simulink model "RATE_ADAPTIVE"  (R2020a)
settings: Solver=FixedStepAuto  StartTime=0.0  StopTime=10.0  FixedStep=1e-3  RelTol=1e-3  EnableMultiTasking=on
undefined symbols (not defined in the file): a, b, c, D0, D1, D10, D11, D12, D13, D2, D3, D4, D5, D6, D7, D8, D9, PTA0, PTA1, PTA2, PTB23, PTB9, PTC16, PTC17, PTC2, PTC3, PTC4, PTD0, PTD1, PTD2, PTD3
libraries: frdmk64flib x16, dspstat3 x1, hdlsllib x1
settings Model: ExtModeTrigDuration=5  Creator=marry  LastModifiedBy=marry
settings OptimizationCC: EnhancedBackFolding=on  PassReuseOutputArgsAs=Individual arguments  ZeroExternalMemoryAtStartup=off  ZeroInternalMemoryAtStartup=off  MaxStackSize=64  OptimizeBlockOrder=speed  DifferentSizesBufferReuse=on  OptimizationCustomize=off  EfficientTunableParamExpr=on
settings DebuggingCC: ParameterTunabilityLossMsg=error
settings HardwareCC: ProdBitPerPointer=32  ProdBitPerSizeT=32  ProdBitPerPtrDiffT=32  ProdLargestAtomicInteger=Long  ProdLargestAtomicFloat=Double  ProdWordSize=32  ProdHWDeviceType=ARM Compatible->ARM Cortex
settings SFSimCC: MATLABDynamicMemAlloc=off
settings RTWCC: SystemTargetFile=ert.tlc  HardwareBoard=NXP FRDM-K64F  TemplateMakefile=ert_default_tmf  Toolchain=GNU Tools for ARM Embedded Processors
settings CodeAppCC: ForceParamTrailComments=on  IgnoreCustomStorageClasses=off  OperatorAnnotations=on  SimulinkDataObjDesc=on  SFDataObjDesc=on  InsertBlockDesc=on

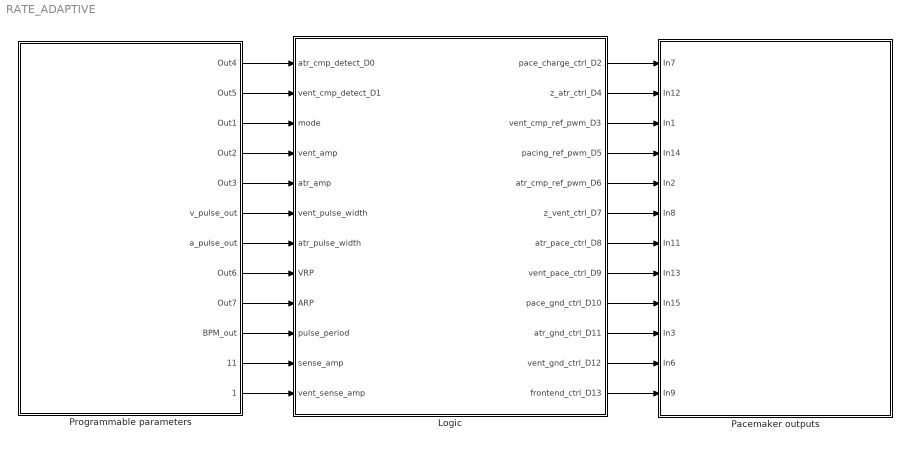
== system RATE_ADAPTIVE ==
  Logic : Stateflow chart  TreatAsAtomicUnit=on
      settings: PortSchema="{\"entries\":[{\"content\":{\"sides\":[{\"content\":{\"connectorIds\":[\"In5\",\"In7\",\"In8\",\"In10\",\"In9\",\"In3\",\"In1\",\"In6\",\"In4\",\"In2\",\"In11\",\"In12\"]},\"type\":\"ConnectorPlacement.EquallySpacedRectSide\",\"uuid\":\"2bdca257-8b9d-4aeb-8f95-3d09a0a4a1f1\"},{\"content\":{\"connectorIds\":[\"Out3\",\"Out8\",\"Out12\",\"Out5\",\"Out11\",\"Out9\",\"Out2\",\"Out7\",\"Out4\",\"Out1\",\"Out6\",\"Out10\"],\"side\":\"RIGHT\"},\"type\":\"ConnectorPlacement.EquallySpacedRectSide\",\"uuid\":\"08f11eea-4805-4115-bb5a-abf58d15e736\"},{\"content\":{\"connectorIds\":[],\"side\":\"TOP\"},\"type\":\"ConnectorPlacement.EquallySpacedRectSide\",\"uuid\":\"37195c58-0653-40fc-a437-a6099f091bb4\"}]},\"type\":\"ConnectorPlacement.EquallySpacedConnector\",\"uuid\":\"b0599c69-dd28-4004-ac14-328e0531830d\"}],\"packageUris\":[\"http://schema.mathworks.com/mf0/Connector/19700101\"],\"version\":\"1.0\"}"
  Pacemaker outputs : Subsystem
  Programmable parameters : Subsystem
  wires:
  Programmable parameters/3(Out1) -> Logic/8(mode)
  Programmable parameters/4(Out2) -> Logic/10(vent_amp)
  Programmable parameters/5(Out3) -> Logic/9(atr_amp)
  Programmable parameters/6(v_pulse_out) -> Logic/3(vent_pulse_width)
  Programmable parameters/7(a_pulse_out) -> Logic/1(atr_pulse_width)
  Programmable parameters/10(BPM_out) -> Logic/2(pulse_period)
  Programmable parameters/9(Out7) -> Logic/4(ARP)
  Programmable parameters/8(Out6) -> Logic/6(VRP)
  Logic/3(pace_charge_ctrl_D2) -> Pacemaker outputs/1(In7)
  Logic/9(z_vent_ctrl_D7) -> Pacemaker outputs/6(In8)
  Logic/2(atr_pace_ctrl_D8) -> Pacemaker outputs/7(In11)
  Logic/7(vent_pace_ctrl_D9) -> Pacemaker outputs/8(In13)
  Logic/4(pace_gnd_ctrl_D10) -> Pacemaker outputs/9(In15)
  Logic/1(atr_gnd_ctrl_D11) -> Pacemaker outputs/10(In3)
  Logic/6(vent_gnd_ctrl_D12) -> Pacemaker outputs/11(In6)
  Logic/10(frontend_ctrl_D13) -> Pacemaker outputs/12(In9)
  Programmable parameters/2(Out5) -> Logic/7(vent_cmp_detect_D1)
  Programmable parameters/1(Out4) -> Logic/5(atr_cmp_detect_D0)
  Logic/8(z_atr_ctrl_D4) -> Pacemaker outputs/2(In12)
  Logic/5(pacing_ref_pwm_D5) -> Pacemaker outputs/4(In14)
  Logic/12(vent_cmp_ref_pwm_D3) -> Pacemaker outputs/3(In1)
  Logic/11(atr_cmp_ref_pwm_D6) -> Pacemaker outputs/5(In2)
  Programmable parameters/11("                                                ") -> Logic/11(sense_amp)
  Programmable parameters/12("                                                1") -> Logic/12(vent_sense_amp)

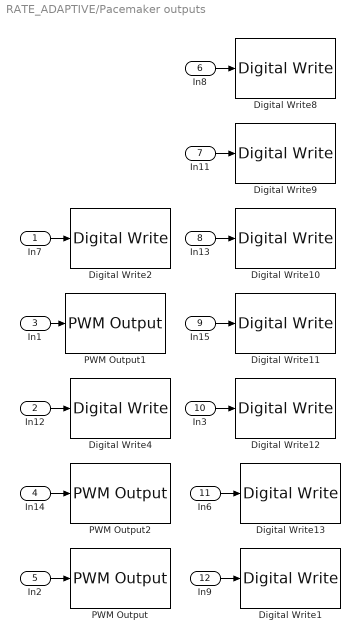
== system RATE_ADAPTIVE/Pacemaker outputs ==
  In7 : Inport
  In12 : Inport  Port=2
  In1 : Inport  Port=3
  In14 : Inport  Port=4
  In2 : Inport  Port=5
  In8 : Inport  Port=6
  In11 : Inport  Port=7
  In13 : Inport  Port=8
  In15 : Inport  Port=9
  In3 : Inport  Port=10
  In6 : Inport  Port=11
  In9 : Inport  Port=12
  Digital Write1 : frdmk64flib/Digital Write  Whichpin=PTD1 (D13)
  Digital Write10 : frdmk64flib/Digital Write  Whichpin=PTC4 (D9)
  Digital Write11 : frdmk64flib/Digital Write  Whichpin=PTD0 (D10)
  Digital Write12 : frdmk64flib/Digital Write  Whichpin=PTD2 (D11)
  Digital Write13 : frdmk64flib/Digital Write  Whichpin=PTD3 (D12)
  Digital Write2 : frdmk64flib/Digital Write  Whichpin=PTB9 (D2)
  Digital Write4 : frdmk64flib/Digital Write  Whichpin=PTB23 (D4)
  Digital Write8 : frdmk64flib/Digital Write  Whichpin=PTC3 (D7)
  Digital Write9 : frdmk64flib/Digital Write  Whichpin=PTA0 (D8)
  PWM Output : frdmk64flib/PWM Output  Whichpin=PTC2 (D6)  InitialFrequency=2000  InitialDutyCycle=0
  PWM Output1 : frdmk64flib/PWM Output  Whichpin=PTA1 (D3)  InitialFrequency=2000  InitialDutyCycle=0
  PWM Output2 : frdmk64flib/PWM Output  Whichpin=PTA2 (D5)  InitialFrequency=2000  InitialDutyCycle=0
  wires:
  In15/1 -> Digital Write11/1
  In12/1 -> Digital Write4/1
  In13/1 -> Digital Write10/1
  In7/1 -> Digital Write2/1
  In14/1 -> PWM Output2/1
  In8/1 -> Digital Write8/1
  In6/1 -> Digital Write13/1
  In11/1 -> Digital Write9/1
  In3/1 -> Digital Write12/1
  In9/1 -> Digital Write1/1
  In1/1 -> PWM Output1/1
  In2/1 -> PWM Output/1

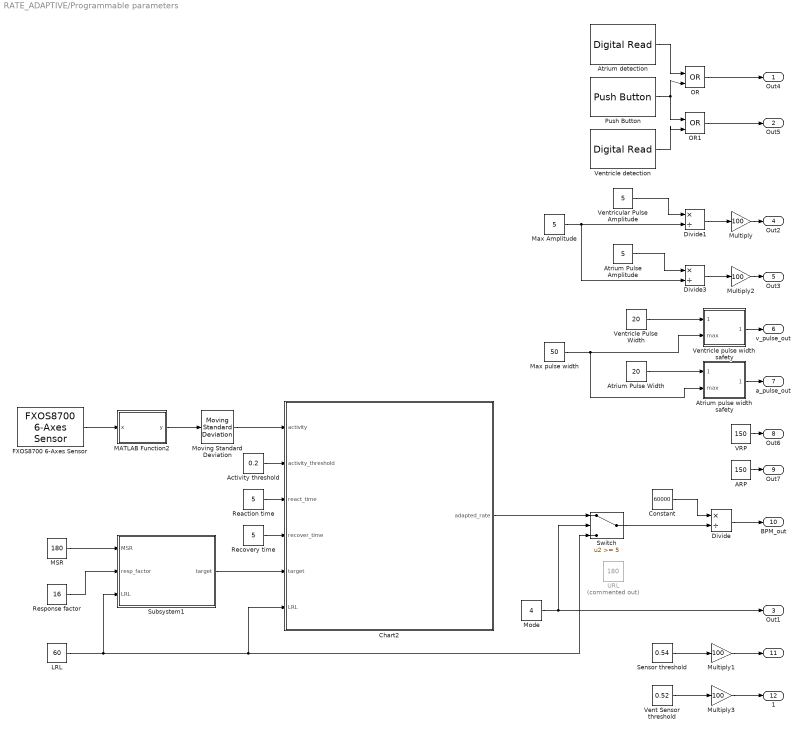
== system RATE_ADAPTIVE/Programmable parameters ==
  ARP : Constant  Value=150
  Activity threshold : Constant  Value=0.2
  Atrium Pulse Amplitude : Constant  Value=5
  Atrium Pulse Width : Constant  Value=20
  Atrium detection : frdmk64flib/Digital Read  Whichpin=PTC16 (D0)  SampleTime=-1
  Atrium pulse width safety : Stateflow chart  TreatAsAtomicUnit=on
  Chart2 : Stateflow chart  TreatAsAtomicUnit=on
      settings: PortSchema="{\"entries\":[{\"content\":{\"sides\":[{\"content\":{\"connectorIds\":[\"In1\",\"In2\",\"In3\",\"In6\",\"In4\",\"In5\"]},\"type\":\"ConnectorPlacement.EquallySpacedRectSide\",\"uuid\":\"bb9994d7-39bc-48cc-973a-fbe19809742a\"},{\"content\":{\"connectorIds\":[\"Out1\"],\"side\":\"RIGHT\"},\"type\":\"ConnectorPlacement.EquallySpacedRectSide\",\"uuid\":\"20773666-cf4d-4804-bbb0-64c8e4eaf526\"},{\"content\":{\"connectorIds\":[],\"side\":\"TOP\"},\"type\":\"ConnectorPlacement.EquallySpacedRectSide\",\"uuid\":\"ef0efbce-984e-4c84-a33f-adc04429966b\"}]},\"type\":\"ConnectorPlacement.EquallySpacedConnector\",\"uuid\":\"39a47510-2469-4520-84cb-e1548f9767a3\"}],\"packageUris\":[\"http://schema.mathworks.com/mf0/Connector/19700101\"],\"version\":\"1.0\"}"
  Constant : Constant  Value=60000
  Divide : Product  Inputs=*/
  Divide1 : Product  Inputs=*/
  Divide3 : Product  Inputs=*/
  FXOS8700 6-Axes Sensor : frdmk64flib/FXOS8700 6-Axes Sensor  Activesensor=Accelerometer only  ODR=100Hz  HybridODR=400Hz  Accelfullrange=-4g to +4g  SampleTime=1/100
  LRL : Constant  Value=60  OutDataTypeStr=uint16
  MATLAB Function2 : MATLAB Function  TreatAsAtomicUnit=on
  MSR : Constant  Value=180  OutDataTypeStr=uint16
  Max Amplitude : Constant  Value=5
  Max pulse width : Constant  Value=50
  Mode : Constant  Value=4
  Moving Standard Deviation : dspstat3/Moving Standard Deviation  Method=Sliding window  ForgettingFactorPort=off  SpecifyWindowLength=on  WindowLength=128  ForgettingFactor=0.9  SimulateUsing=Code generation
      settings: SourceProductBaseCode=DS
  Multiply{,1..3} (4 alike) : Gain  Gain=100
  OR : Logic  Operator=OR  IconShape=distinctive  AllPortsSameDT=off  OutDataTypeStr=boolean
  OR1 : Logic  Operator=OR  IconShape=distinctive  AllPortsSameDT=off  OutDataTypeStr=boolean
  Push Button : frdmk64flib/Push Button  Whichswitch=SW2  SampleTime1=-1
  Reaction time : Constant  Value=5
  Recovery time : Constant  Value=5
  Response factor : Constant  Value=16  OutDataTypeStr=uint16
  Sensor threshold : Constant  Value=0.54
  Subsystem1 : Subsystem
  Switch : Switch  Threshold=5
  URL : Constant  Commented=on  Value=180
  VRP : Constant  Value=150
  Vent Sensor threshold : Constant  Value=0.52
  Ventricle Pulse Width : Constant  Value=20
  "Ventricle detection " : frdmk64flib/Digital Read  Whichpin=PTC17 (D1)  SampleTime=-1
  Ventricle pulse width safety : Stateflow chart  TreatAsAtomicUnit=on
  Ventricular Pulse Amplitude : Constant  Value=5
  Out4 : Outport
  Out5 : Outport  Port=2
  Out1 : Outport  Port=3
  Out2 : Outport  Port=4
  Out3 : Outport  Port=5
  v_pulse_out : Outport  Port=6
  a_pulse_out : Outport  Port=7
  Out6 : Outport  Port=8
  Out7 : Outport  Port=9
  BPM_out : Outport  Port=10
  "                                                " : Outport  Port=11
  "                                                1" : Outport  Port=12
  wires:
  Max Amplitude/1 -> Divide3/2, Divide1/2
  Ventricular Pulse Amplitude/1 -> Divide1/1
  Atrium Pulse Width/1 -> Atrium pulse width safety/1(pulse_in)
  Atrium Pulse Amplitude/1 -> Divide3/1
  Max pulse width/1 -> Ventricle pulse width safety/2(max), Atrium pulse width safety/2(max)
  ARP/1 -> Out7/1
  Divide1/1 -> Multiply/1
  Divide3/1 -> Multiply2/1
  Ventricle Pulse Width/1 -> Ventricle pulse width safety/1(pulse_in)
  Multiply/1 -> Out2/1
  Multiply2/1 -> Out3/1
  VRP/1 -> Out6/1
  Ventricle pulse width safety/1(v_pulse_out) -> v_pulse_out/1
  Atrium pulse width safety/1(a_pulse_out) -> a_pulse_out/1
  "Ventricle detection "/1 -> OR1/2
  Atrium detection/1 -> OR/1
  Push Button/1 -> OR1/1, OR/2
  OR1/1 -> Out5/1
  OR/1 -> Out4/1
  Multiply1/1 -> "                                                "/1
  Sensor threshold/1 -> Multiply1/1
  Vent Sensor threshold/1 -> Multiply3/1
  Multiply3/1 -> "                                                1"/1
  Reaction time/1 -> Chart2/3(react_time)
  Chart2/1(adapted_rate) -> Switch/1
  Activity threshold/1 -> Chart2/2(activity_threshold)
  Response factor/1 -> Subsystem1/2(resp_factor)
  FXOS8700 6-Axes Sensor/1 -> MATLAB Function2/1(x)
  Subsystem1/1(target) -> Chart2/4(target)
  Recovery time/1 -> Chart2/6(recover_time)
  Mode/1 -> Out1/1, Switch/2
  Moving Standard Deviation/1 -> Chart2/1(activity)
  MSR/1 -> Subsystem1/1(MSR)
  MATLAB Function2/1(y) -> Moving Standard Deviation/1
  LRL/1 -> Switch/3, Chart2/5(LRL), Subsystem1/3(LRL)
  Switch/1 -> Divide/2
  Constant/1 -> Divide/1
  Divide/1 -> BPM_out/1

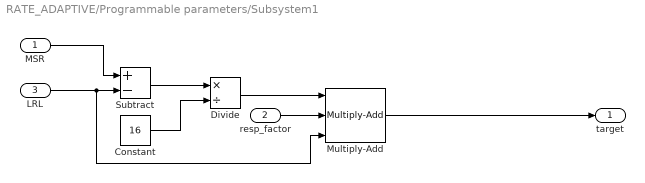
== system RATE_ADAPTIVE/Programmable parameters/Subsystem1 ==
  MSR : Inport
  resp_factor : Inport  Port=2
  LRL : Inport  Port=3
  Constant : Constant  Value=16
  Divide : Product  Inputs=*/
  Multiply-Add : hdlsllib/HDL Operations/Multiply-Add  Function=c+(a.*b)  datatype=uint16  RndMeth=Nearest  DoSatur=off  FMA=off
      settings: SourceProductBaseCode=SL
  Subtract : Sum  Inputs=+-
  target : Outport  OutDataTypeStr=uint16  SourceOfInitialOutputValue=Input signal
  wires:
  MSR/1 -> Subtract/1
  LRL/1 -> Multiply-Add/3, Subtract/2
  Subtract/1 -> Divide/1
  Constant/1 -> Divide/2
  Divide/1 -> Multiply-Add/1
  resp_factor/1 -> Multiply-Add/2
  Multiply-Add/1 -> target/1

== stateflow chart RATE_ADAPTIVE/Programmable parameters/Atrium pulse width safety ==
  state Acceptable
    entry:
    a_pulse_out = pulse_in;
  state Entry
  state Unacceptable
    entry:
    a_pulse_out = max;
  Entry -> Acceptable [order 1] : [pulse_in <= max || pulse_in > 0]
  (default) -> Entry
  Entry -> Unacceptable [order 2]
  data: pulse_in input; max input; a_pulse_out output

== stateflow chart RATE_ADAPTIVE/Programmable parameters/Ventricle pulse width safety ==
  state Acceptable
    entry:
    v_pulse_out = pulse_in;
  state Entry
  state Unacceptable
    entry:
    v_pulse_out = max;
  Entry -> Acceptable [order 1] : [pulse_in <= max || pulse_in > 0]
  (default) -> Entry
  Entry -> Unacceptable [order 2]
  data: pulse_in input; max input; v_pulse_out output

== stateflow chart RATE_ADAPTIVE/Logic ==
  state AAI
    state AAI_Pacing
      entry:
      frontend_ctrl_D13= 0;
      pace_charge_ctrl_D2 = 0;
      pace_gnd_ctrl_D10= 1;
      atr_pace_ctrl_D8 = 1;
      atr_gnd_ctrl_D11= 0;
      z_atr_ctrl_D4= 0;
    state AAI_Charging
      entry:
      frontend_ctrl_D13= 1;
      pacing_ref_pwm_D5= atr_amp;
      atr_pace_ctrl_D8 = 0;
      pace_charge_ctrl_D2 = 1;
      pace_gnd_ctrl_D10= 1;
      atr_gnd_ctrl_D11= 1;
      atr_cmp_ref_pwm_D6= sense_amp;
      z_atr_ctrl_D4= 0;
    state AAI_Inhibition
      entry:
      frontend_ctrl_D13= 0;
      atr_pace_ctrl_D8 = 0;
      atr_gnd_ctrl_D11= 1;
      pace_charge_ctrl_D2 = 1;
      pace_gnd_ctrl_D10= 1;
      z_atr_ctrl_D4= 0;
    (default) -> AAI_Charging
    AAI_Charging -> AAI.AAI_Pacing [order 2] : after(pulse_period - atr_pulse_width - ARP,msec)
    AAI_Charging -> (junction 113) [order 1] : [atr_cmp_detect_D0 == 1]
    (junction 113) -> AAI.AAI_Inhibition : [after(atr_pulse_width,msec)]
    AAI.AAI_Pacing -> AAI.AAI_Inhibition : [after(atr_pulse_width,msec)]
    AAI.AAI_Inhibition -> AAI_Charging : [after(ARP, msec)]
  state VOO
    state VOO_Charging
      entry:
      vent_pace_ctrl_D9 = 0;
      pacing_ref_pwm_D5= vent_amp;
      pace_charge_ctrl_D2 = 1;
      pace_gnd_ctrl_D10= 1;
      vent_gnd_ctrl_D12= 1;
      z_vent_ctrl_D7 = 0;
    state VOO_Pacing
      entry:
      pace_charge_ctrl_D2 = 0;
      pace_gnd_ctrl_D10= 1;
      vent_pace_ctrl_D9 = 1;
      vent_gnd_ctrl_D12 = 0;
      z_vent_ctrl_D7 = 0;
    (default) -> VOO_Charging
    VOO_Charging -> VOO_Pacing : [after(pulse_period - vent_pulse_width,msec)]
    VOO_Pacing -> VOO_Charging : [after(vent_pulse_width,msec)]
  state VVI
    state VVI_Charging
      entry:
      frontend_ctrl_D13= 1;
      pacing_ref_pwm_D5= vent_amp;
      vent_pace_ctrl_D9 = 0;
      pace_charge_ctrl_D2 = 1;
      pace_gnd_ctrl_D10= 1;
      vent_gnd_ctrl_D12= 1;
      vent_cmp_ref_pwm_D3= vent_sense_amp;
      z_vent_ctrl_D7= 0;
    state VVI_Pacing
      entry:
      frontend_ctrl_D13= 0;
      pace_charge_ctrl_D2 = 0;
      pace_gnd_ctrl_D10= 1;
      vent_pace_ctrl_D9 = 1;
      vent_gnd_ctrl_D12= 0;
      z_vent_ctrl_D7= 0;
    state VVI_Inhibition
      entry:
      frontend_ctrl_D13= 0;
      vent_pace_ctrl_D9 = 0;
      vent_gnd_ctrl_D12= 1;
      pace_charge_ctrl_D2 = 1;
      pace_gnd_ctrl_D10= 1;
      z_vent_ctrl_D7= 0;
    (default) -> VVI_Charging
    VVI_Charging -> VVI.VVI_Pacing [order 2] : after(pulse_period - vent_pulse_width - VRP,msec)
    VVI_Charging -> (junction 148) [order 1] : [vent_cmp_detect_D1 == 1]
    (junction 148) -> VVI.VVI_Inhibition : [after(vent_pulse_width,msec)]
    VVI.VVI_Pacing -> VVI.VVI_Inhibition : [after(vent_pulse_width,msec)]
    VVI.VVI_Inhibition -> VVI_Charging : [after(VRP, msec)]
  state Start
  state AOO
    state AOO_Charging
      entry:
      atr_pace_ctrl_D8 = 0;
      pacing_ref_pwm_D5= atr_amp;
      pace_charge_ctrl_D2 = 1;
      pace_gnd_ctrl_D10= 1;
      atr_gnd_ctrl_D11= 1;
      z_atr_ctrl_D4= 0;
    state AOO_Pacing
      entry:
      pace_charge_ctrl_D2 = 0;
      pace_gnd_ctrl_D10= 1;
      atr_pace_ctrl_D8 = 1;
      atr_gnd_ctrl_D11= 0;
      z_atr_ctrl_D4= 0;
    (default) -> AOO_Charging
    AOO_Charging -> AOO_Pacing : [after(pulse_period - atr_pulse_width,msec)]
    AOO_Pacing -> AOO_Charging : [after(atr_pulse_width,msec)]
  state AAIR
    state AAI_Pacing
      %Discharging C22 into Atrium
      entry:
      pace_charge_ctrl_D2 = 0;
      pace_gnd_ctrl_D10= 1;
      atr_pace_ctrl_D8 = 1;
      atr_gnd_ctrl_D11= 0;
      z_atr_ctrl_D4 = 0;
      z_vent_ctrl_D7 = 0;
      vent_gnd_ctrl_D12 = 0;
      vent_pace_ctrl_D9 = 0;
    state AAIR_Charging
      entry:
      %sensing circuitry
      frontend_ctrl_D13= 1;
      %PWM Threshold
      atr_cmp_ref_pwm_D6= sense_amp;
      vent_cmp_ref_pwm_D3 = 0;
      %charging C22
      atr_pace_ctrl_D8 = 0;
      vent_pace_ctrl_D9 = 0;
      pacing_ref_pwm_D5= atr_amp;
      pace_charge_ctrl_D2 = 1;
      %discharge C21 Capacitor
      pace_gnd_ctrl_D10= 1;
      vent_pace_ctrl_D9 = 0;
      z_atr_ctrl_D4 = 0;
      z_vent_ctrl_D7 = 0;
      atr_pace_ctrl_D8 = 0;
      atr_gnd_ctrl_D11= 1;
      vent_gnd_ctrl_D12 = 0;
    state AAI_Inhibition
      entry:
      %Discharge C21 Capacitor
      pace_gnd_ctrl_D10= 1;
      vent_pace_ctrl_D9 = 0;
      z_atr_ctrl_D4 = 0;
      z_vent_ctrl_D7 = 0;
      frontend_ctrl_D13= 0;
      atr_pace_ctrl_D8 = 0;
      atr_gnd_ctrl_D11= 1;
      vent_gnd_ctrl_D12 = 0;
      %Charge C22
      atr_pace_ctrl_D8 = 0;
      vent_pace_ctrl_D9 = 0;
      pacing_ref_pwm_D5= atr_amp;
      pace_charge_ctrl_D2 = 1;
    (default) -> AAIR_Charging
    AAIR_Charging -> AAIR.AAI_Pacing [order 1] : [after(pulse_period - atr_pulse_width - ARP,msec)]
    AAIR_Charging -> (junction 161) [order 2] : [atr_cmp_detect_D0 == 1]
    (junction 161) -> AAIR.AAI_Inhibition : [after(atr_pulse_width,msec)]
    AAIR.AAI_Pacing -> AAIR.AAI_Inhibition : [after(atr_pulse_width,msec)]
    AAIR.AAI_Inhibition -> AAIR_Charging : [after(ARP, msec)]
  state VVIR
    state VVI_Pacing
      %Discharging C22 into Atrium
      entry:
      pace_charge_ctrl_D2 = 0;
      pace_gnd_ctrl_D10= 1;
      atr_pace_ctrl_D8 = 0;
      atr_gnd_ctrl_D11= 0;
      z_atr_ctrl_D4 = 0;
      z_vent_ctrl_D7 = 0;
      vent_gnd_ctrl_D12 = 0;
      vent_pace_ctrl_D9 = 1;
    state VVIR_Charging
      entry:
      %sensing circuitry
      frontend_ctrl_D13= 1;
      %PWM Threshold
      atr_cmp_ref_pwm_D6= 0;
      vent_cmp_ref_pwm_D3 = vent_sense_amp;
      %charging C22
      atr_pace_ctrl_D8 = 0;
      vent_pace_ctrl_D9 = 0;
      pacing_ref_pwm_D5= vent_amp;
      pace_charge_ctrl_D2 = 1;
      %discharge C21 Capacitor
      pace_gnd_ctrl_D10= 1;
      vent_pace_ctrl_D9 = 0;
      z_atr_ctrl_D4 = 0;
      z_vent_ctrl_D7 = 0;
      atr_pace_ctrl_D8 = 0;
      atr_gnd_ctrl_D11= 1;
      vent_gnd_ctrl_D12 = 0;
    state VVI_Inhibition
      entry:
      %Discharge C21 Capacitor
      pace_gnd_ctrl_D10= 1;
      vent_pace_ctrl_D9 = 0;
      z_atr_ctrl_D4 = 0;
      z_vent_ctrl_D7 = 0;
      frontend_ctrl_D13= 0;
      atr_pace_ctrl_D8 = 0;
      atr_gnd_ctrl_D11=0;
      vent_gnd_ctrl_D12 = 1;
      %Charge C22
      atr_pace_ctrl_D8 = 0;
      vent_pace_ctrl_D9 = 0;
      pacing_ref_pwm_D5= vent_amp;
      pace_charge_ctrl_D2 = 1;
    (default) -> VVIR_Charging
    VVIR_Charging -> VVIR.VVI_Pacing [order 1] : [after(pulse_period - atr_pulse_width - VRP,msec)]
    VVIR_Charging -> (junction 168) [order 2] : [vent_cmp_detect_D1 == 1]
    (junction 168) -> VVIR.VVI_Inhibition : [after(vent_pulse_width,msec)]
    VVIR.VVI_Pacing -> VVIR.VVI_Inhibition : [after(vent_pulse_width,msec)]
    VVIR.VVI_Inhibition -> VVIR_Charging : [after(VRP, msec)]
  Start -> AAI [order 3] : [mode == 3]
  AAI -> Start : [mode ~= 3]
  VOO -> Start : [mode ~= 2]
  VVI -> Start : [mode ~= 4]
  Start -> VOO [order 2] : [mode == 2]
  Start -> VVI [order 4] : [mode == 4]
  (default) -> Start
  Start -> AOO [order 1] : [mode == 1]
  Start -> AAIR [order 5] : [mode == 5]
  AAIR -> Start : [mode ~= 5]
  AOO -> Start : [mode ~= 1]
  Start -> VVIR [order 6] : [mode == 6]
  VVIR -> Start : [mode ~= 6]
  data: atr_pulse_width input; pulse_period input; atr_gnd_ctrl_D11 output; atr_pace_ctrl_D8 output; pace_charge_ctrl_D2 output; pace_gnd_ctrl_D10 output; pacing_ref_pwm_D5 output; vent_gnd_ctrl_D12 output; vent_pace_ctrl_D9 output; z_atr_ctrl_D4 output; z_vent_ctrl_D7 output; vent_pulse_width input; ARP input; frontend_ctrl_D13 output; atr_cmp_detect_D0 input; VRP input; vent_cmp_detect_D1 input; mode input; atr_amp input; vent_amp input; atr_cmp_ref_pwm_D6 output; vent_cmp_ref_pwm_D3 output; sense_amp input; vent_sense_amp input

== stateflow chart RATE_ADAPTIVE/Programmable parameters/Chart2 ==
  state Active
    entry:
    adapted_rate = adapted_rate + inc;
  state Target
    entry:
    adapted_rate = target;
  state Start
    entry:
    inc = ceil((target - LRL) / react_time);
    dec = ceil((target - LRL) / recover_time);
    adapted_rate = LRL;
  state Error
    entry:
    adapted_rate = adapted_rate - inc;
  state Resting
    entry:
    adapted_rate = adapted_rate - dec;
  Target -> Target [order 2] : [activity >= activity_threshold]
  Active -> Active [order 1] : after(1000,msec)[adapted_rate <= target]
  (default) -> Start
  Active -> Target [order 3] : [adapted_rate > target]
  Start -> Active [order 1] : [activity >= activity_threshold]
  Start -> Start [order 2] : [activity < activity_threshold]
  Active -> Error [order 2] : [activity < activity_threshold]
  Error -> Active [order 1] : [activity >= activity_threshold]
  Resting -> Active [order 3] : [activity >= activity_threshold]
  Target -> Resting [order 1] : [activity < activity_threshold]
  Resting -> Start [order 1] : [adapted_rate <= LRL]
  Error -> Resting [order 2] : [after(1000,msec)]
  Resting -> Resting [order 2] : after(1000, msec)[adapted_rate > LRL]
  data: activity input; activity_threshold input double; react_time input; target input; adapted_rate output uint16; dec local uint16; inc local uint16; LRL input uint16; recover_time input

== matlab function RATE_ADAPTIVE/Programmable parameters/MATLAB Function2 ==
  data: x input; y output
function y = avg_accel(x)
y = sqrt(x(1)^2 + x(2)^2 + x(3)^2);
